simulink model "mchp_acim_dsPIC33A"  (R2025b)
settings: Solver=FixedStepDiscrete  StartTime=0.0  StopTime=25  FixedStep=Ts  RelTol=1e-3  EnableMultiTasking=on
values from neighbouring files (symbols this model uses):
  dataType = 'single'    [mchp_acim_foc_dsPIC33A_data.m]
  PWM_frequency = 20e3    (= 20000)    [mchp_acim_foc_dsPIC33A_data.m]
  PWM_frequency_mc = PWM_frequency    (= 20000)    [mchp_acim_foc_dsPIC33A_data.m]
  SpeedFilterCutoff = 40    [mchp_acim_foc_dsPIC33A_data.m]
  Ts = T_pwm    (= 5e-05)    [mchp_acim_foc_dsPIC33A_data.m]
  Ts_mc = T_pwm_mc    (= 5e-05)    [mchp_acim_foc_dsPIC33A_data.m]
  Ts_motor = T_pwm_mc    (= 5e-05)    [mchp_acim_foc_dsPIC33A_data.m]
  Ts_serialIn = 100e-3    (= 0.1)    [mchp_acim_foc_dsPIC33A_data.m]
undefined symbols (not defined in the file or in its folder): A0, A4, acim, ADC, appState, B0, C10, C11, C6, C7, C8, CS_param, D11, D12, DiscIntNeverNeededParam, estim_pll, estim_qei, inverter, Max, MaxPer, ms, NumBits1, NumBits2, P1, P17, P20, P39, P40, P41, P43, P44, P60, P61, PI_params_SI, Pin, PWM4_Trg1, Resol, s, target, us, VmaxPhase
libraries: simulink x47, MCHP_Blockset x24, mcbcontrolslib x5, mcbeeMathTransformLib x4, slpidlib x4, svdutilitieslib x1, autolibim x1, mcbplantlib x1
(part 6 of 6)

== system mchp_acim_dsPIC33A/Control algorithm/Motor Control Application/FOC/PI_Controller_Speed ==
  N_ref : Inport
  N_fb : Inport  Port=2
  Reset : Inport  Port=3
  Discrete PI Controller with anti-windup & reset : slpidlib/PID Controller  Controller=PI  Form=Parallel  TimeDomain=Discrete-time  UseExternalTs=off  SampleTime=Ts_mc  IntegratorMethod=Forward Euler  FilterMethod=Forward Euler  ControllerParametersSource=external  P=1  I=1  UseKiTs=on  D=0  UseExternalDerivativeSource=off  N=100  UseFilter=on  TunerSelectOption=Transfer Function Based (PID Tuner App)  InitialConditionSource=external  InitialConditionForIntegrator=0  InitialConditionForFilter=0  DifferentiatorICPrevScaledInput=0  ExternalReset=rising  TrackingMode=off  Kt=1  LimitOutput=on  SatLimitsSource=internal  UpperSaturationLimit=acim.Iq0  LowerSaturationLimit=-acim.Iq0  LinearizeAsGain=on  AntiWindupMode=clamping  Kb=1  LimitIntegrator=on  UpperIntegratorSaturationLimit=acim.Iq0  LowerIntegratorSaturationLimit=-acim.Iq0  RndMeth=Simplest  POutMin=[]  POutMax=[]  IOutMin=[]  IOutMax=[]  DOutMin=[]  DOutMax=[]  NOutMin=[]  NOutMax=[]  SumOutMin=[]  SumOutMax=[]  SaturationOutDataTypeStr=Inherit: Inherit via back propagation  SaturationOutMin=[]  SaturationOutMax=[]  PParamMin=[]  PParamMax=[]  IParamMin=[]  IParamMax=[]  DParamMin=[]  DParamMax=[]  NParamMin=[]  NParamMax=[]  KbParamMin=[]  KbParamMax=[]  KtParamMin=[]  KtParamMax=[]  KbOutMin=[]  KbOutMax=[]  KtOutMin=[]  KtOutMax=[]  IntegratorOutMin=[]  IntegratorOutMax=[]  FilterOutMin=[]  FilterOutMax=[]  SumI1OutMin=[]  SumI1OutMax=[]  SumI2OutMin=[]  SumI2OutMax=[]  SumI3OutMin=[]  SumI3OutMax=[]  SumI4OutMin=[]  SumI4OutMax=[]  SumDOutMin=[]  SumDOutMax=[]  DifferentiatorOutMin=[]  DifferentiatorOutMax=[]  FilterDiffOutCoefMin=[]  FilterDiffOutCoefMax=[]  ReciprocalOutMin=[]  ReciprocalOutMax=[]  SumDenOutMin=[]  SumDenOutMax=[]  SumNumOutMin=[]  SumNumOutMax=[]  DivideOutMin=[]  DivideOutMax=[]  UdiffTsProdOutMin=[]  UdiffTsProdOutMax=[]  NTsProdOutMin=[]  NTsProdOutMax=[]  UintegralTsProdOutMin=[]  UintegralTsProdOutMax=[]  UngainTsProdOutMin=[]  UngainTsProdOutMax=[]  ClampingZeroOutDataTypeStr=Inherit: Inherit via back propagation  ClampingZeroOutMin=[]  ClampingZeroOutMax=[]  FilterDenConstantOutDataTypeStr=Inherit: Inherit via back propagation  FilterDenConstantOutMin=[]  FilterDenConstantOutMax=[]  PCopyOutDataTypeStr=Inherit: Inherit via back propagation  PCopyOutMin=[]  PCopyOutMax=[]  NCopyOutDataTypeStr=Inherit: Inherit via back propagation  NCopyOutMin=[]  NCopyOutMax=[]  IntegratorContinuousStateAttributes=''  IntegratorStateMustResolveToSignalObject=off  IntegratorRTWStateStorageClass=Auto  FilterContinuousStateAttributes=''  FilterStateMustResolveToSignalObject=off  FilterRTWStateStorageClass=Auto  ParallelPVariant=ExternalParameters  IdealPVariant=Disabled  IVariant=ExternalParameters  DVariant=Disabled  IntegratorVariant=Discrete  SatVariant=Enabled  AWVariant=DiscClampingParallel  PCopyVariant=Disabled  TRVariant=Disabled  FdbkBlocksVariant=Forward  IdealPFdbkVariant=Disabled  SatFdbkVariant=Disabled  DerivativeFilterVariant=Disabled  NVariant=Disabled  NCopyVariant=Disabled_SignalSpec  FilterICVariant=Disabled  IntegratorICVariant=ExternalICs  ExternalResetVariant=ExternalReset  TRSumVariant=Passthrough  SumFdbkVariant=Disabled  SumVariant=Sum_PI  TsampFilterVariant=InternalTs  TsampNgainVariant=Passthrough  TsampIntegralVariant=Disabled_SignalSpec  ExternalSaturationOutDataTypeStr=Inherit: Same as second input  DerivativeSourceVariant=Disabled  PreIntVariant=InternalPreInt
  Ki1 : Constant  Value=PI_params_SI.Ki_speed*Ts_mc  OutDataTypeStr=single  SampleTime=Ts_mc
  Kp1 : Constant  Value=PI_params_SI.Kp_speed  OutDataTypeStr=single  SampleTime=Ts_mc
  Sum : Sum  Inputs=|+-  OutDataTypeStr=Inherit: Same as first input
  Iq_ref : Outport  VectorParamsAs1DForOutWhenUnconnected=off
  wires:
  N_ref/1 -> Sum/1
  [Integrator_PI_Speed] -> Discrete PI Controller with anti-windup & reset/5
  Reset/1 -> Discrete PI Controller with anti-windup & reset/4
  Sum/1 -> Discrete PI Controller with anti-windup & reset/1
  N_fb/1 -> Sum/2
  Kp1/1 -> Discrete PI Controller with anti-windup & reset/2
  Ki1/1 -> Discrete PI Controller with anti-windup & reset/3
  Discrete PI Controller with anti-windup & reset/1 -> Iq_ref/1

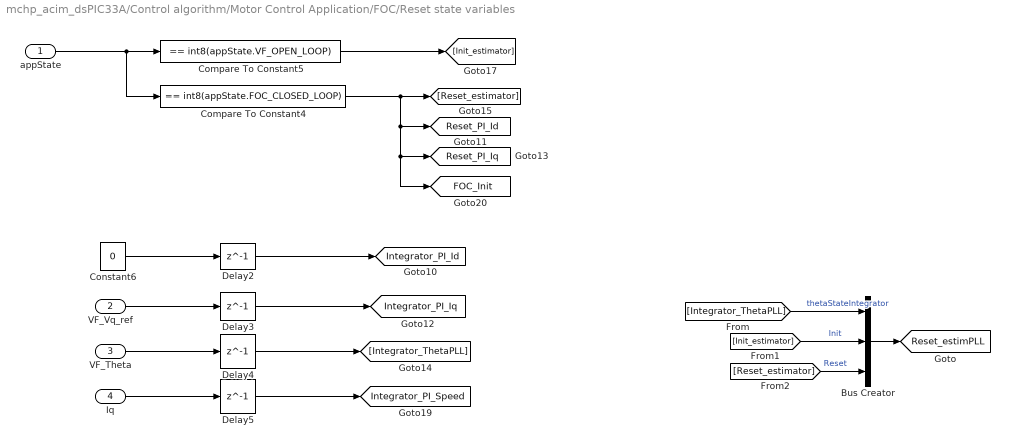
== system mchp_acim_dsPIC33A/Control algorithm/Motor Control Application/FOC/Reset state variables ==
  appState : Inport
  VF_Vq_ref : Inport  Port=2
  VF_Theta : Inport  Port=3
  Iq : Inport  Port=4
  Bus Creator : BusCreator  Inputs=3
  Compare To Constant4 : simulink/Logic and Bit Operations/Compare To Constant  relop===  const=int8(appState.FOC_CLOSED_LOOP)  OutDataTypeStr=boolean
  Compare To Constant5 : simulink/Logic and Bit Operations/Compare To Constant  relop===  const=int8(appState.VF_OPEN_LOOP)  OutDataTypeStr=boolean
  Constant6 : Constant  Value=0  OutDataTypeStr=single  SampleTime=-1
  Delay{2..5} (4 alike) : Delay  DelayLength=1
  tag scope: FOC_Init=global, Integrator_PI_Id=global, Integrator_PI_Iq=global, Integrator_PI_Speed=global, Reset_PI_Id=global, Reset_PI_Iq=global, Reset_estimPLL=global
  wires:
  Constant6/1 -> Delay2/1
  Compare To Constant4/1 -> [FOC_Init], [Reset_PI_Iq], [Reset_PI_Id], [Reset_estimator]
  Delay5/1 -> [Integrator_PI_Speed]
  Delay3/1 -> [Integrator_PI_Iq]
  Iq/1 -> Delay5/1
  appState/1 -> Compare To Constant4/1, Compare To Constant5/1
  VF_Theta/1 -> Delay4/1
  VF_Vq_ref/1 -> Delay3/1
  Delay2/1 -> [Integrator_PI_Id]
  Delay4/1 -> [Integrator_ThetaPLL]
  Compare To Constant5/1 -> [Init_estimator]
  [Integrator_ThetaPLL] -> Bus Creator/1  "thetaStateIntegrator"
  [Init_estimator] -> Bus Creator/2  "Init"
  [Reset_estimator] -> Bus Creator/3  "Reset"
  Bus Creator/1 -> [Reset_estimPLL]

== system mchp_acim_dsPIC33A/Control algorithm/Motor Control Application/FOC/VbyF ControlReference ==
  Reset : Inport
  speedRef : Inport  Port=2
  Enable : EnablePort
  Gain : Gain  Gain=(2*pi*acim.p/60)*Ts_mc  OutDataTypeStr=single
  Position Generator : mcbcontrolslib/Position Generator  AngleOutput=Radians  InitialThetaSource=Specify via dialog  ExternalReset=active high resets to initial condition  Offset=0
  Saturation : Saturate  UpperLimit=acim.V_rated*sqrt(2/3)*0.9  LowerLimit=10
  VbyF_constant : Gain  Gain=CS_param.VbyF_constant
  Wrap_to_pi1 : Subsystem  VariantControl=VSS_STD
  OL_Theta : Outport
  V_ref : Outport  Port=2
  wires:
  Gain/1 -> Position Generator/1
  Position Generator/1 -> Wrap_to_pi1/1(θ)  "Theta_in"
  Reset/1 -> Position Generator/2
  Wrap_to_pi1/1(θ (-π,π)) -> OL_Theta/1
  speedRef/1 -> VbyF_constant/1, Gain/1
  VbyF_constant/1 -> Saturation/1
  Saturation/1 -> V_ref/1

== system mchp_acim_dsPIC33A/Control algorithm/Motor Control Application/appState State Machine/Speed Ramp_limiter ==
  Reset_trigger : Inport
  Initial_value : Inport  Port=2
  Target_speed : Inport  Port=3
  stop : Inport  Port=4
  Compare To Constant2 : simulink/Logic and Bit Operations/Compare To Constant  relop=>=  const=CS_param.SpeedRampRate  OutDataTypeStr=boolean
  Compare To Constant7 : simulink/Logic and Bit Operations/Compare To Constant  relop=<=  const=-CS_param.SpeedRampRate  OutDataTypeStr=boolean
  Constant1 : Constant  Value=acim.N_min/2  OutDataTypeStr=single  SampleTime=-1
  Constant10 : Constant  Value=-CS_param.SpeedRampRate  OutDataTypeStr=single  SampleTime=-1
  Constant9 : Constant  Value=CS_param.SpeedRampRate  OutDataTypeStr=single  SampleTime=-1
  Delay1 : Delay  DelayLength=1  InitialConditionSource=Input port  InitialCondition=-1  ExternalReset=Level
      settings: InputPortMap=u0,r5,p4
  Product1 : Product
  Product3 : Product
  Subtract2 : Sum  Inputs=+-
  Subtract4 : Sum  Inputs=+++
  Switch : Switch  Criteria=u2 > Threshold  SaturateOnIntegerOverflow=off  InputSameDT=off
  Reference_Speed : Outport
  wires:
  Constant9/1 -> Product1/1
  Compare To Constant7/1 -> Product3/2
  Subtract2/1 -> Compare To Constant7/1, Compare To Constant2/1
  Delay1/1 -> Subtract2/2, Reference_Speed/1, Subtract4/1
  Constant10/1 -> Product3/1
  Compare To Constant2/1 -> Product1/2
  Subtract4/1 -> Delay1/1
  Product3/1 -> Subtract4/3
  Product1/1 -> Subtract4/2
  Reset_trigger/1 -> Delay1/2
  Switch/1 -> Subtract2/1
  Initial_value/1 -> Delay1/3
  stop/1 -> Switch/2
  Target_speed/1 -> Switch/3
  Constant1/1 -> Switch/1

== system mchp_acim_dsPIC33A/Inverter and Motor model/Simulation/Motor and Inverter/Inverter ==
  Duty_abc : Inport
  Average-Value Inverter : mcbplantlib/Average-Value Inverter
  Constant2 : Constant  Value=inverter.V_dc  OutDataTypeStr=single  SampleTime=-1
  Data Type Conversion1 : DataTypeConversion  OutDataTypeStr=single  RndMeth=Simplest  SaturateOnIntegerOverflow=off
  Vabc : Outport  VectorParamsAs1DForOutWhenUnconnected=off
  wires:
  Constant2/1 -> Average-Value Inverter/2
  Data Type Conversion1/1 -> Average-Value Inverter/1
  Duty_abc/1 -> Data Type Conversion1/1
  Average-Value Inverter/1 -> Vabc/1  "Vabc"

== system mchp_acim_dsPIC33A/MCHV-230VAC-1.5kW Development Board dsPIC33AK128MC106 MC DIM/Center & sign reversal1/Moving Average/Enabled Subsystem1 ==
  In1 : Inport
  Enable : EnablePort  ZeroCross=off
  Out1 : Outport
  wires:
  In1/1 -> Out1/1

== system mchp_acim_dsPIC33A/Control algorithm/Data Monitoring/SerialOutDrivers/codegen/SCI_Tx ==
  note: Fast Serial Data Monitoring (32-bit)
  Data_Log : Inport
  Constant : Constant  Value=target.frameSize -1  OutDataTypeStr=uint16
  Counter Limited : simulink/Sources/Counter Limited  uplimit=target.frameSize-1  tsamp=-1
  Data : Subsystem  TreatAsAtomicUnit=on
  Data Type Conversion : DataTypeConversion  OutDataTypeStr=uint16  RndMeth=Simplest  SaturateOnIntegerOverflow=off
  End : Subsystem  TreatAsAtomicUnit=on
  If : If  NumInputs=2  IfExpression=u1 == 0  ElseIfExpressions=u1 == u2
  Start : Subsystem  TreatAsAtomicUnit=on
  wires:
  If/3 -> Data/Action
  Counter Limited/1 -> Data Type Conversion/1
  If/2 -> End/Action
  If/1 -> Start/Action
  Data_Log/1 -> End/1(Data), Start/1(Data), Data/1(Data)
  Constant/1 -> If/2
  Data Type Conversion/1 -> If/1

== system mchp_acim_dsPIC33A/Control algorithm/Data Monitoring/Subsystem/Data_Conditioning_Tx/Data_Type_Fixed_Point ==
  In1 : Inport
  Data Type Conversion : DataTypeConversion  OutDataTypeStr=fixdt(1,32,28)  RndMeth=Simplest  SaturateOnIntegerOverflow=off
  Data Type Conversion3 : DataTypeConversion  OutDataTypeStr=uint32  ConvertRealWorld=Stored Integer (SI)  RndMeth=Simplest  SaturateOnIntegerOverflow=off
  Data_Log : Outport
  wires:
  In1/1 -> Data Type Conversion/1
  Data Type Conversion3/1 -> Data_Log/1
  Data Type Conversion/1 -> Data Type Conversion3/1

== system mchp_acim_dsPIC33A/Control algorithm/Data Monitoring/Subsystem/Data_Conditioning_Tx/Data_Type_Float ==
  In1 : Inport
  Byte Pack : svdutilitieslib/Byte Pack  maskPackedDataType=uint8  datatypes={'single'}  byteAlign=4  blockPlatform=tic2000
  Data_Log : Outport
  wires:
  Byte Pack/1 -> Data_Log/1
  In1/1 -> Byte Pack/1

== system mchp_acim_dsPIC33A/Control algorithm/Data Monitoring/Variant Subsystem/Codegen/Extract User inputs ==
  SCi_Data : Inport
  Bitwise OR : simulink/Logic and Bit Operations/Bitwise Operator  logicop=OR  UseBitMask=off  NumInputPorts=2  BitMask=bin2dec('11011001')  BitMaskRealWorld=Stored Integer
  Data Type Conversion1 : DataTypeConversion  OutDataTypeStr=uint16  RndMeth=Simplest  SaturateOnIntegerOverflow=off
  Data Type Conversion2 : DataTypeConversion  OutDataTypeStr=int16  ConvertRealWorld=Stored Integer (SI)  RndMeth=Simplest  SaturateOnIntegerOverflow=off
  Data Type Conversion3 : DataTypeConversion  OutDataTypeStr=uint16  RndMeth=Simplest  SaturateOnIntegerOverflow=off
  Data Type Conversion4 : DataTypeConversion  OutDataTypeStr=dataType  RndMeth=Simplest  SaturateOnIntegerOverflow=off
  Demux : Demux  Outputs=8
  RPM to rad/s : Gain  Gain=pi/30  RndMeth=Simplest  OutDataTypeStr=Inherit: Same as input
  Shift Arithmetic : ArithShift  BitShiftNumber=-8
  Terminator{,1..3} (4 alike) : Terminator
  Enable : Outport
  SpeedRef : Outport  Port=2
  DebugSel : Outport  Port=3
  wires:
  Demux/3 -> Enable/1
  Data Type Conversion2/1 -> Data Type Conversion4/1  "SpeedRef"
  Demux/4 -> DebugSel/1
  Bitwise OR/1 -> Data Type Conversion2/1
  Demux/1 -> Data Type Conversion1/1
  SCi_Data/1 -> Demux/1
  Shift Arithmetic/1 -> Bitwise OR/2
  Data Type Conversion3/1 -> Shift Arithmetic/1
  Data Type Conversion1/1 -> Bitwise OR/1
  Demux/7 -> Terminator2/1
  Demux/2 -> Data Type Conversion3/1
  Demux/5 -> Terminator/1
  Demux/6 -> Terminator1/1
  Demux/8 -> Terminator3/1
  RPM to rad/s/1 -> SpeedRef/1  "SpeedRef"
  Data Type Conversion4/1 -> RPM to rad/s/1

== system mchp_acim_dsPIC33A/Control algorithm/Motor Control Application/FOC/Current_Controllers/Dynamic Limit ==
  Vd : Inport
  Constant : Constant  Value=CS_param.VmaxPhase  OutDataTypeStr=single  SampleTime=-1
  Product : Product  RndMeth=Simplest  OutDataTypeStr=Inherit: Same as first input
  Product1 : Product  RndMeth=Simplest  OutDataTypeStr=Inherit: Same as first input
  Saturation : Saturate  UpperLimit=CS_param.VmaxPhase^2  LowerLimit=0
  Sqrt : Sqrt  RndMeth=Simplest
  Sum1 : Sum  Inputs=+-|  RndMeth=Simplest  OutDataTypeStr=Inherit: Same as first input
  Vq_max : Outport
  wires:
  Vd/1 -> Product/1, Product/2
  Product/1 -> Saturation/1
  Constant/1 -> Product1/2, Product1/1
  Saturation/1 -> Sum1/2
  Sum1/1 -> Sqrt/1
  Product1/1 -> Sum1/1
  Sqrt/1 -> Vq_max/1

== system mchp_acim_dsPIC33A/Control algorithm/Motor Control Application/FOC/Current_Controllers/PI_Controller_Id ==
  I_ref : Inport
  I_fb : Inport  Port=2
  Discrete PI Controller with anti-windup & reset : slpidlib/PID Controller  Controller=PI  Form=Parallel  TimeDomain=Discrete-time  UseExternalTs=off  SampleTime=Ts_mc  IntegratorMethod=Forward Euler  FilterMethod=Forward Euler  ControllerParametersSource=external  P=1  I=1  UseKiTs=on  D=0  UseExternalDerivativeSource=off  N=100  UseFilter=on  TunerSelectOption=Transfer Function Based (PID Tuner App)  InitialConditionSource=external  InitialConditionForIntegrator=0  InitialConditionForFilter=0  DifferentiatorICPrevScaledInput=0  ExternalReset=rising  TrackingMode=off  Kt=1  LimitOutput=on  SatLimitsSource=internal  UpperSaturationLimit=CS_param.VmaxPhase  LowerSaturationLimit=-CS_param.VmaxPhase  LinearizeAsGain=on  AntiWindupMode=clamping  Kb=1  LimitIntegrator=on  UpperIntegratorSaturationLimit=CS_param.VmaxPhase  LowerIntegratorSaturationLimit=-CS_param.VmaxPhase  RndMeth=Simplest  POutMin=[]  POutMax=[]  IOutMin=[]  IOutMax=[]  DOutMin=[]  DOutMax=[]  NOutMin=[]  NOutMax=[]  SumOutMin=[]  SumOutMax=[]  SaturationOutDataTypeStr=Inherit: Inherit via back propagation  SaturationOutMin=[]  SaturationOutMax=[]  PParamMin=[]  PParamMax=[]  IParamMin=[]  IParamMax=[]  DParamMin=[]  DParamMax=[]  NParamMin=[]  NParamMax=[]  KbParamMin=[]  KbParamMax=[]  KtParamMin=[]  KtParamMax=[]  KbOutMin=[]  KbOutMax=[]  KtOutMin=[]  KtOutMax=[]  IntegratorOutMin=[]  IntegratorOutMax=[]  FilterOutMin=[]  FilterOutMax=[]  SumI1OutMin=[]  SumI1OutMax=[]  SumI2OutMin=[]  SumI2OutMax=[]  SumI3OutMin=[]  SumI3OutMax=[]  SumI4OutMin=[]  SumI4OutMax=[]  SumDOutMin=[]  SumDOutMax=[]  DifferentiatorOutMin=[]  DifferentiatorOutMax=[]  FilterDiffOutCoefMin=[]  FilterDiffOutCoefMax=[]  ReciprocalOutMin=[]  ReciprocalOutMax=[]  SumDenOutMin=[]  SumDenOutMax=[]  SumNumOutMin=[]  SumNumOutMax=[]  DivideOutMin=[]  DivideOutMax=[]  UdiffTsProdOutMin=[]  UdiffTsProdOutMax=[]  NTsProdOutMin=[]  NTsProdOutMax=[]  UintegralTsProdOutMin=[]  UintegralTsProdOutMax=[]  UngainTsProdOutMin=[]  UngainTsProdOutMax=[]  ClampingZeroOutDataTypeStr=Inherit: Inherit via back propagation  ClampingZeroOutMin=[]  ClampingZeroOutMax=[]  FilterDenConstantOutDataTypeStr=Inherit: Inherit via back propagation  FilterDenConstantOutMin=[]  FilterDenConstantOutMax=[]  PCopyOutDataTypeStr=Inherit: Inherit via back propagation  PCopyOutMin=[]  PCopyOutMax=[]  NCopyOutDataTypeStr=Inherit: Inherit via back propagation  NCopyOutMin=[]  NCopyOutMax=[]  IntegratorContinuousStateAttributes=''  IntegratorStateMustResolveToSignalObject=off  IntegratorRTWStateStorageClass=Auto  FilterContinuousStateAttributes=''  FilterStateMustResolveToSignalObject=off  FilterRTWStateStorageClass=Auto  ParallelPVariant=ExternalParameters  IdealPVariant=Disabled  IVariant=ExternalParameters  DVariant=Disabled  IntegratorVariant=Discrete  SatVariant=Enabled  AWVariant=DiscClampingParallel  PCopyVariant=Disabled  TRVariant=Disabled  FdbkBlocksVariant=Forward  IdealPFdbkVariant=Disabled  SatFdbkVariant=Disabled  DerivativeFilterVariant=Disabled  NVariant=Disabled  NCopyVariant=Disabled_SignalSpec  FilterICVariant=Disabled  IntegratorICVariant=ExternalICs  ExternalResetVariant=ExternalReset  TRSumVariant=Passthrough  SumFdbkVariant=Disabled  SumVariant=Sum_PI  TsampFilterVariant=InternalTs  TsampNgainVariant=Passthrough  TsampIntegralVariant=Disabled_SignalSpec  ExternalSaturationOutDataTypeStr=Inherit: Same as second input  DerivativeSourceVariant=Disabled  PreIntVariant=InternalPreInt
  Ki3 : Constant  Value=PI_params_SI.Ki_i*Ts_mc  OutDataTypeStr=single  SampleTime=Ts_mc
  Kp2 : Constant  Value=PI_params_SI.Kp_i  OutDataTypeStr=single  SampleTime=Ts_mc
  Sum : Sum  Inputs=|+-  OutDataTypeStr=Inherit: Same as first input
  V_ref : Outport  VectorParamsAs1DForOutWhenUnconnected=off
  wires:
  [Integrator_PI_Id] -> Discrete PI Controller with anti-windup & reset/5
  Sum/1 -> Discrete PI Controller with anti-windup & reset/1
  Discrete PI Controller with anti-windup & reset/1 -> V_ref/1
  I_fb/1 -> Sum/2
  I_ref/1 -> Sum/1
  Ki3/1 -> Discrete PI Controller with anti-windup & reset/3
  Kp2/1 -> Discrete PI Controller with anti-windup & reset/2
  [Reset_PI_Id] -> Discrete PI Controller with anti-windup & reset/4

== system mchp_acim_dsPIC33A/Control algorithm/Motor Control Application/FOC/Current_Controllers/PI_Controller_Iq ==
  I_ref : Inport
  I_fb : Inport  Port=2
  Vq_max : Inport  Port=3
  Discrete PI Controller with anti-windup & reset : slpidlib/PID Controller  Controller=PI  Form=Parallel  TimeDomain=Discrete-time  UseExternalTs=off  SampleTime=Ts_mc  IntegratorMethod=Forward Euler  FilterMethod=Forward Euler  ControllerParametersSource=external  P=1  I=1  UseKiTs=on  D=0  UseExternalDerivativeSource=off  N=100  UseFilter=on  TunerSelectOption=Transfer Function Based (PID Tuner App)  InitialConditionSource=external  InitialConditionForIntegrator=0  InitialConditionForFilter=0  DifferentiatorICPrevScaledInput=0  ExternalReset=rising  TrackingMode=off  Kt=1  LimitOutput=on  SatLimitsSource=external  UpperSaturationLimit=VmaxPhase  LowerSaturationLimit=-VmaxPhase  LinearizeAsGain=on  AntiWindupMode=clamping  Kb=1  LimitIntegrator=on  UpperIntegratorSaturationLimit=CS_param.VmaxPhase  LowerIntegratorSaturationLimit=-CS_param.VmaxPhase  RndMeth=Simplest  POutMin=[]  POutMax=[]  IOutMin=[]  IOutMax=[]  DOutMin=[]  DOutMax=[]  NOutMin=[]  NOutMax=[]  SumOutMin=[]  SumOutMax=[]  SaturationOutDataTypeStr=Inherit: Inherit via back propagation  SaturationOutMin=[]  SaturationOutMax=[]  PParamMin=[]  PParamMax=[]  IParamMin=[]  IParamMax=[]  DParamMin=[]  DParamMax=[]  NParamMin=[]  NParamMax=[]  KbParamMin=[]  KbParamMax=[]  KtParamMin=[]  KtParamMax=[]  KbOutMin=[]  KbOutMax=[]  KtOutMin=[]  KtOutMax=[]  IntegratorOutMin=[]  IntegratorOutMax=[]  FilterOutMin=[]  FilterOutMax=[]  SumI1OutMin=[]  SumI1OutMax=[]  SumI2OutMin=[]  SumI2OutMax=[]  SumI3OutMin=[]  SumI3OutMax=[]  SumI4OutMin=[]  SumI4OutMax=[]  SumDOutMin=[]  SumDOutMax=[]  DifferentiatorOutMin=[]  DifferentiatorOutMax=[]  FilterDiffOutCoefMin=[]  FilterDiffOutCoefMax=[]  ReciprocalOutMin=[]  ReciprocalOutMax=[]  SumDenOutMin=[]  SumDenOutMax=[]  SumNumOutMin=[]  SumNumOutMax=[]  DivideOutMin=[]  DivideOutMax=[]  UdiffTsProdOutMin=[]  UdiffTsProdOutMax=[]  NTsProdOutMin=[]  NTsProdOutMax=[]  UintegralTsProdOutMin=[]  UintegralTsProdOutMax=[]  UngainTsProdOutMin=[]  UngainTsProdOutMax=[]  ClampingZeroOutDataTypeStr=Inherit: Inherit via back propagation  ClampingZeroOutMin=[]  ClampingZeroOutMax=[]  FilterDenConstantOutDataTypeStr=Inherit: Inherit via back propagation  FilterDenConstantOutMin=[]  FilterDenConstantOutMax=[]  PCopyOutDataTypeStr=Inherit: Inherit via back propagation  PCopyOutMin=[]  PCopyOutMax=[]  NCopyOutDataTypeStr=Inherit: Inherit via back propagation  NCopyOutMin=[]  NCopyOutMax=[]  IntegratorContinuousStateAttributes=''  IntegratorStateMustResolveToSignalObject=off  IntegratorRTWStateStorageClass=Auto  FilterContinuousStateAttributes=''  FilterStateMustResolveToSignalObject=off  FilterRTWStateStorageClass=Auto  ParallelPVariant=ExternalParameters  IdealPVariant=Disabled  IVariant=ExternalParameters  DVariant=Disabled  IntegratorVariant=Discrete  SatVariant=External  AWVariant=DiscClampingParallel  PCopyVariant=Disabled  TRVariant=Disabled  FdbkBlocksVariant=Forward  IdealPFdbkVariant=Disabled  SatFdbkVariant=Disabled  DerivativeFilterVariant=Disabled  NVariant=Disabled  NCopyVariant=Disabled_SignalSpec  FilterICVariant=Disabled  IntegratorICVariant=ExternalICs  ExternalResetVariant=ExternalReset  TRSumVariant=Passthrough  SumFdbkVariant=Disabled  SumVariant=Sum_PI  TsampFilterVariant=InternalTs  TsampNgainVariant=Passthrough  TsampIntegralVariant=Disabled_SignalSpec  ExternalSaturationOutDataTypeStr=Inherit: Same as second input  DerivativeSourceVariant=Disabled  PreIntVariant=InternalPreInt
  Gain : Gain  Gain=-1
  Ki3 : Constant  Value=PI_params_SI.Ki_i*Ts_mc  OutDataTypeStr=single  SampleTime=Ts_mc
  Kp2 : Constant  Value=PI_params_SI.Kp_i  OutDataTypeStr=single  SampleTime=Ts_mc
  Sum : Sum  Inputs=|+-  OutDataTypeStr=Inherit: Same as first input
  V_ref : Outport  VectorParamsAs1DForOutWhenUnconnected=off
  wires:
  [Integrator_PI_Iq] -> Discrete PI Controller with anti-windup & reset/5
  Sum/1 -> Discrete PI Controller with anti-windup & reset/1
  I_ref/1 -> Sum/1
  I_fb/1 -> Sum/2
  Discrete PI Controller with anti-windup & reset/1 -> V_ref/1
  [Reset_PI_Iq] -> Discrete PI Controller with anti-windup & reset/4
  Kp2/1 -> Discrete PI Controller with anti-windup & reset/2
  Ki3/1 -> Discrete PI Controller with anti-windup & reset/3
  Gain/1 -> Discrete PI Controller with anti-windup & reset/7
  Vq_max/1 -> Discrete PI Controller with anti-windup & reset/6, Gain/1

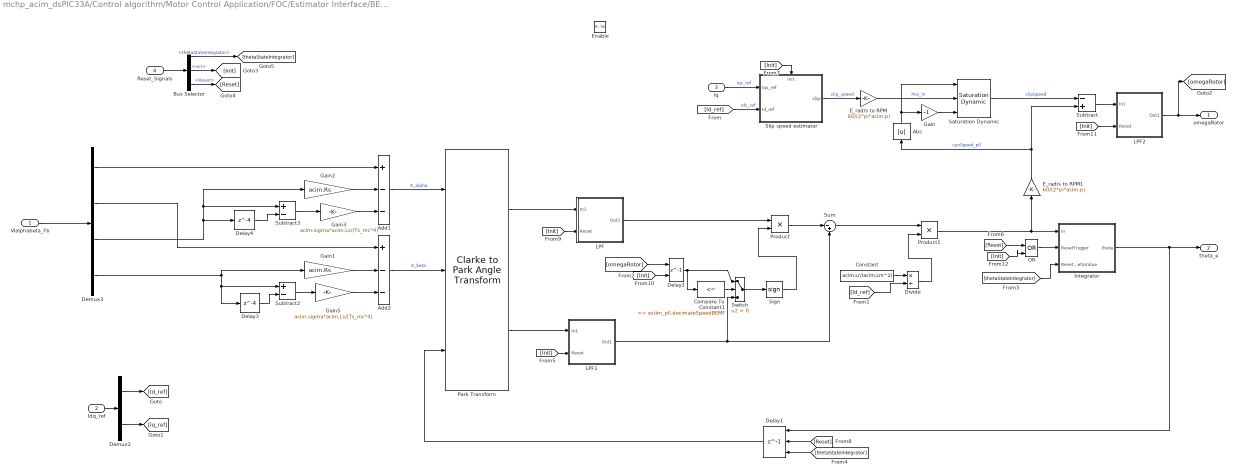
== system mchp_acim_dsPIC33A/Control algorithm/Motor Control Application/FOC/Estimator Interface/BEMF-PLL Sensorless estimator1 ==
  VIalphabeta_Fb : Inport
  Idq_ref : Inport  Port=2
  Iq : Inport  Port=3
  Reset_Signals : Inport  Port=4
  Enable : EnablePort
  Abs : Abs  SaturateOnIntegerOverflow=off
  Add1 : Sum  Inputs=+--
  Add2 : Sum  Inputs=+--
  Bus Selector : BusSelector  OutputSignals=thetaStateIntegrator,Init,Reset
  Compare To Constant1 : simulink/Logic and Bit Operations/Compare To Constant  relop=<=  const=estim_pll.decimateSpeedBEMF  OutDataTypeStr=boolean
  Constant : Constant  Value=acim.Lr/(acim.Lm^2)  OutDataTypeStr=single  SampleTime=-1
  Delay1 : Delay  DelayLength=1  InitialConditionSource=Input port  ExternalReset=Rising
      settings: InputPortMap=u0,r5,p4
  Delay2 : Delay  DelayLength=1  ExternalReset=Rising
      settings: InputPortMap=u0,r5
  Delay3 : Delay  DelayLength=4
  Delay4 : Delay  DelayLength=4
  Demux2 : Demux  Outputs=2
  Demux3 : Demux
  Divide : Product  Inputs=*/
  E_rad/s to RPM : Gain  Gain=60/(2*pi*acim.p)  RndMeth=Simplest  OutDataTypeStr=Inherit: Same as input
  E_rad/s to RPM1 : Gain  Gain=60/(2*pi*acim.p)  RndMeth=Simplest  OutDataTypeStr=Inherit: Same as input
  Gain : Gain  Gain=-1
  Gain1 : Gain  Gain=acim.Rs  OutDataTypeStr=Inherit: Same as input
  Gain2 : Gain  Gain=acim.Rs  OutDataTypeStr=Inherit: Same as input
  Gain3 : Gain  Gain=acim.sigma*acim.Ls/(Ts_mc*4)  OutDataTypeStr=single
  Gain5 : Gain  Gain=acim.sigma*acim.Ls/(Ts_mc*4)  OutDataTypeStr=single
  Integrator : Subsystem
  LPF : Subsystem
  LPF1 : Subsystem
  LPF2 : Subsystem
  OR : Logic  Operator=OR  IconShape=distinctive  AllPortsSameDT=off  OutDataTypeStr=boolean
  Park Transform : mcbeeMathTransformLib/Clarke to Park Angle Transform  AxisAlignment=D-axis  UseWithEmbedded=on  PhaseInput=Two inputs  ThetaInput=Electrical position  AngleInput=Radians  N_points=1024
      settings: LibrarySourceBlock=mcbcontrolslib/Park Transform
  Product : Product
  Product1 : Product
  Saturation Dynamic : simulink/Discontinuities/Saturation Dynamic  OutMin=[]  OutMax=[]  OutDataTypeStr=Inherit: Same as second input  OutDataType=fixdt(1, 16)  OutScaling=2^-10  DoSatur=off
  Sign : Signum
  Slip speed estimator : Subsystem
      settings: PortSchema="{\"entries\":[{\"content\":{\"sides\":[{\"content\":{\"connectorIds\":[\"In1\",\"In2\"]},\"type\":\"ConnectorPlacement.EquallySpacedRectSide\",\"uuid\":\"981370cc-fd81-43b0-8526-c66c0de54492\"},{\"content\":{\"connectorIds\":[\"Out1\"],\"side\":\"RIGHT\"},\"type\":\"ConnectorPlacement.EquallySpacedRectSide\",\"uuid\":\"4a494ed1-db1f-498e-bde6-92ddc00b959f\"},{\"content\":{\"connectorIds\":[\"In3\"],\"side\":\"TOP\"},\"type\":\"ConnectorPlacement.EquallySpacedRectSide\",\"uuid\":\"ae0cfd30-3876-4cea-9557-00c7dbe354cc\"}]},\"type\":\"ConnectorPlacement.EquallySpacedConnector\",\"uuid\":\"0c170fee-798a-45d3-abb0-c7a31b583370\"}],\"packageUris\":[\"http://schema.mathworks.com/mf0/Connector/R2020b\"],\"version\":\"1.0\"}"
  Subtract : Sum  Inputs=-+
  Subtract2 : Sum  Inputs=+-
  Subtract3 : Sum  Inputs=+-
  Sum : Sum  Inputs=|-+
  Switch : Switch  Criteria=u2 > Threshold  SaturateOnIntegerOverflow=off  InputSameDT=off
  omegaRotor : Outport
  theta_e : Outport  Port=2
  wires:
  Sign/1 -> Product/2
  Sum/1 -> Product1/1
  Delay1/1 -> Park Transform/3
  Add2/1 -> Park Transform/2  "E_beta"
  Product/1 -> Sum/1
  VIalphabeta_Fb/1 -> Demux3/1
  Add1/1 -> Park Transform/1  "E_alpha"
  Park Transform/1 -> LPF/1(In1)
  LPF/1(Out1) -> Product/1
  Park Transform/2 -> LPF1/1(In1)
  Integrator/1(theta) -> Delay1/1, theta_e/1
  Idq_ref/1 -> Demux2/1
  Demux2/1 -> [Id_ref]
  Demux2/2 -> [Iq_ref]
  Constant/1 -> Divide/1
  [Id_ref] -> Divide/2
  Divide/1 -> Product1/2
  Iq/1 -> Slip speed estimator/1(Iqs_ref)  "Iqs_ref"
  Slip speed estimator/1(slip) -> E_rad/s to RPM/1  "slip_speed"
  E_rad/s to RPM/1 -> Saturation Dynamic/2  "Pos_In"
  Product1/1 -> Integrator/1(In), E_rad/s to RPM1/1
  LPF2/1(Out1) -> [omegaRotor], omegaRotor/1
  E_rad/s to RPM1/1 -> Abs/1, Subtract/2  "synSpeed_pll"
  Gain/1 -> Saturation Dynamic/3
  Saturation Dynamic/1 -> Subtract/1  "slipSpeed"
  Compare To Constant1/1 -> Switch/2
  Delay2/1 -> Compare To Constant1/1, Switch/1
  LPF1/1(Out1) -> Switch/3, Sum/2
  Switch/1 -> Sign/1
  OR/1 -> Integrator/2(ResetTrigger)
  [Id_ref] -> Slip speed estimator/2(Id_ref)  "Ids_ref"
  Abs/1 -> Saturation Dynamic/1, Gain/1
  Subtract/1 -> LPF2/1(In1)
  Demux3/1 -> Add1/1
  Demux3/3 -> Delay4/1, Gain2/1, Subtract3/1
  Subtract3/1 -> Gain3/1
  Delay4/1 -> Subtract3/2
  Gain2/1 -> Add1/2
  Gain3/1 -> Add1/3
  Gain5/1 -> Add2/3
  Delay3/1 -> Subtract2/2
  Subtract2/1 -> Gain5/1
  Demux3/2 -> Add2/1
  Demux3/4 -> Gain1/1, Subtract2/1, Delay3/1
  Gain1/1 -> Add2/2
  [omegaRotor] -> Delay2/1
  [Reset] -> OR/1
  [Init] -> OR/2
  Reset_Signals/1 -> Bus Selector/1
  Bus Selector/2 -> [Init]  "<Init>"
  Bus Selector/3 -> [Reset]  "<Reset>"
  Bus Selector/1 -> [thetaStateIntegrator]  "<thetaStateIntegrator>"
  [thetaStateIntegrator] -> Integrator/3(ResetThetaValue)
  [thetaStateIntegrator] -> Delay1/3
  [Reset] -> Delay1/2
  [Init] -> LPF1/2(Reset)
  [Init] -> LPF/2(Reset)
  [Init] -> Delay2/2
  [Init] -> LPF2/2(Reset)
  [Init] -> Slip speed estimator/3(Init)

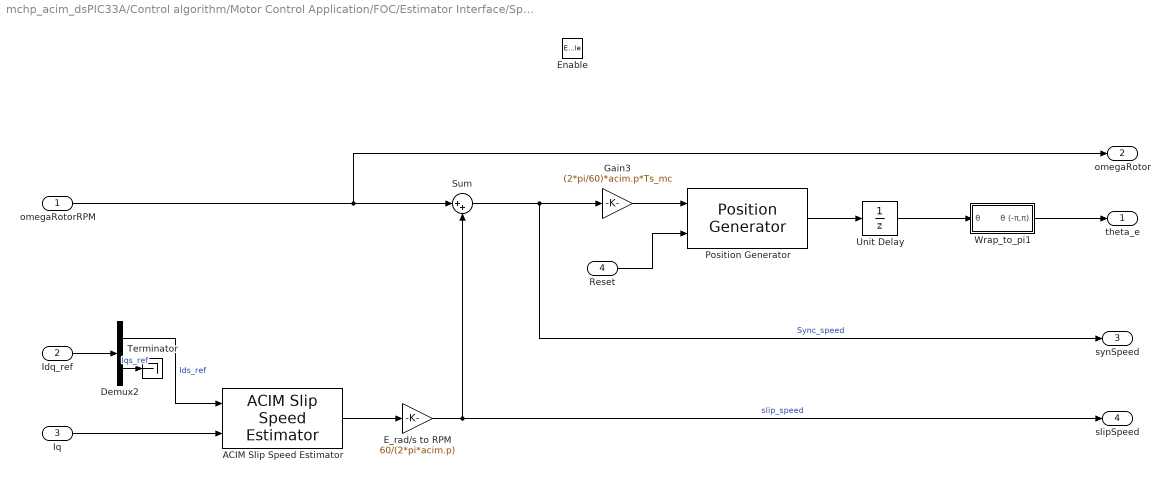
== system mchp_acim_dsPIC33A/Control algorithm/Motor Control Application/FOC/Estimator Interface/Speed & postion interface (sensored) ==
  omegaRotorRPM : Inport
  Idq_ref : Inport  Port=2
  Iq : Inport  Port=3
  Reset : Inport  Port=4
  Enable : EnablePort
  ACIM Slip Speed Estimator : mcbcontrolslib/ACIM Slip Speed Estimator  polePairs=acim.p  Rr=acim.Rr  Llr=acim.Llr  Lm=acim.Lm  N_sat=acim.N_rated/20  Units=SI Units  N_base=acim.N_base
  Demux2 : Demux  Outputs=2
  E_rad/s to RPM : Gain  Gain=60/(2*pi*acim.p)  RndMeth=Simplest  OutDataTypeStr=Inherit: Same as input
  Gain3 : Gain  Gain=(2*pi/60)*acim.p*Ts_mc  RndMeth=Simplest  OutDataTypeStr=Inherit: Same as input
  Position Generator : mcbcontrolslib/Position Generator  AngleOutput=Radians  InitialThetaSource=Specify via dialog  ExternalReset=active high resets to initial condition  Offset=0
  Sum : Sum  Inputs=|++
  Terminator : Terminator
  Unit Delay : UnitDelay  SampleTime=-1  HasFrameUpgradeWarning=on
  Wrap_to_pi1 : Subsystem  VariantControl=VSS_STD
  theta_e : Outport
  omegaRotor : Outport  Port=2
  synSpeed : Outport  Port=3
  slipSpeed : Outport  Port=4
  wires:
  Position Generator/1 -> Unit Delay/1
  Sum/1 -> synSpeed/1, Gain3/1  "Sync_speed"
  Demux2/1 -> ACIM Slip Speed Estimator/1  "Ids_ref"
  ACIM Slip Speed Estimator/1 -> E_rad/s to RPM/1
  Gain3/1 -> Position Generator/1
  Reset/1 -> Position Generator/2
  Idq_ref/1 -> Demux2/1
  Unit Delay/1 -> Wrap_to_pi1/1(θ)
  omegaRotorRPM/1 -> omegaRotor/1, Sum/1
  E_rad/s to RPM/1 -> Sum/2, slipSpeed/1  "slip_speed"
  Wrap_to_pi1/1(θ (-π,π)) -> theta_e/1
  Iq/1 -> ACIM Slip Speed Estimator/2
  Demux2/2 -> Terminator/1  "Iqs_ref"

== system mchp_acim_dsPIC33A/Control algorithm/Motor Control Application/FOC/Generate Id reference/Enabled Subsystem ==
  In1 : Inport
  Enable : EnablePort
  Out1 : Outport
  wires:
  In1/1 -> Out1/1

== system mchp_acim_dsPIC33A/Control algorithm/Motor Control Application/FOC/Generate Id reference/Inverse Speed based Flux Weakening ==
  SpeedRef : Inport
  Enable : EnablePort
  Compare To Constant : simulink/Logic and Bit Operations/Compare To Constant  relop=>=  const=acim.N_rated/2  OutDataTypeStr=uint8
  If : If  IfExpression=(u1 > 0)
  If Action Subsystem : Subsystem  TreatAsAtomicUnit=on
  If Action Subsystem1 : Subsystem  TreatAsAtomicUnit=on
  Merge : Merge
  Id_ref : Outport
  wires:
  SpeedRef/1 -> If Action Subsystem/1(speedRef), Compare To Constant/1
  Compare To Constant/1 -> If/1
  If Action Subsystem/1(id_ref) -> Merge/1
  If/1 -> If Action Subsystem/Action
  If/2 -> If Action Subsystem1/Action
  If Action Subsystem1/1(id_ref) -> Merge/2
  Merge/1 -> Id_ref/1

== system mchp_acim_dsPIC33A/Control algorithm/Motor Control Application/FOC/Generate Id reference/OffsetRamp ==
  In1 : Inport
  In2 : Inport  Port=2
  Abs2 : Abs  SaturateOnIntegerOverflow=off
  Compare To Constant6 : simulink/Logic and Bit Operations/Compare To Constant  relop=<=  const=CS_param.currentRampRate  OutDataTypeStr=boolean
  Constant14 : Constant  Value=CS_param.currentRampRate  OutDataTypeStr=single
  Constant6 : Constant  Value=0  OutDataTypeStr=single
  Delay : Delay  DelayLength=1  InitialConditionSource=Input port  InitialCondition=-1  ExternalReset=Rising
      settings: InputPortMap=u0,r5,p4
  Product2 : Product
  Sign2 : Signum
  Subtract3 : Sum  Inputs=+-  OutDataTypeStr=single  AccumDataTypeStr=single
  Switch1 : Switch  Criteria=u2 > Threshold  SaturateOnIntegerOverflow=off  InputSameDT=off
  Out1 : Outport
  wires:
  Subtract3/1 -> Delay/1, Switch1/3, Abs2/1
  Constant6/1 -> Switch1/1
  Sign2/1 -> Product2/1
  Delay/1 -> Sign2/1, Subtract3/1
  Abs2/1 -> Compare To Constant6/1
  Product2/1 -> Subtract3/2
  Constant14/1 -> Product2/2
  Compare To Constant6/1 -> Switch1/2
  Switch1/1 -> Out1/1
  In1/1 -> Delay/2
  In2/1 -> Delay/3

== system mchp_acim_dsPIC33A/Control algorithm/Motor Control Application/FOC/Generate Id reference/Voltage limit based Flux Weakening ==
  SpeedRef : Inport
  vdq : Inport  Port=2
  Enable : EnablePort
  Add1 : Sum
  Compare To Constant : simulink/Logic and Bit Operations/Compare To Constant  relop=<=  const=acim.N_rated/2  OutDataTypeStr=boolean
  Constant : Constant  Value=CS_param.VmaxPhase*0.9  OutDataTypeStr=single
  Delay One Step : Delay  DelayLength=1
  Demux : Demux  Outputs=2
  Discrete PID Controller : slpidlib/PID Controller  Controller=PI  Form=Parallel  TimeDomain=Discrete-time  UseExternalTs=off  SampleTime=-1  IntegratorMethod=Forward Euler  FilterMethod=Forward Euler  ControllerParametersSource=internal  P=PI_params_SI.Kp_FW  I=PI_params_SI.Ki_FW  UseKiTs=on  D=0  UseExternalDerivativeSource=off  N=100  UseFilter=on  TunerSelectOption=Transfer Function Based (PID Tuner App)  InitialConditionSource=internal  InitialConditionForIntegrator=acim.Id0  InitialConditionForFilter=0  DifferentiatorICPrevScaledInput=0  ExternalReset=level  TrackingMode=off  Kt=1  LimitOutput=on  SatLimitsSource=internal  UpperSaturationLimit=acim.Id0  LowerSaturationLimit=acim.Id0/2  LinearizeAsGain=off  AntiWindupMode=none  Kb=1  LimitIntegrator=on  UpperIntegratorSaturationLimit=acim.Id0  LowerIntegratorSaturationLimit=acim.Id0/2  POutMin=[]  POutMax=[]  IOutMin=[]  IOutMax=[]  DOutMin=[]  DOutMax=[]  NOutMin=[]  NOutMax=[]  SumOutMin=[]  SumOutMax=[]  SaturationOutMin=[]  SaturationOutMax=[]  PParamMin=[]  PParamMax=[]  IParamMin=[]  IParamMax=[]  DParamMin=[]  DParamMax=[]  NParamMin=[]  NParamMax=[]  KbParamMin=[]  KbParamMax=[]  KtParamMin=[]  KtParamMax=[]  KbOutMin=[]  KbOutMax=[]  KtOutMin=[]  KtOutMax=[]  IntegratorOutMin=[]  IntegratorOutMax=[]  FilterOutMin=[]  FilterOutMax=[]  SumI1OutMin=[]  SumI1OutMax=[]  SumI2OutMin=[]  SumI2OutMax=[]  SumI3OutMin=[]  SumI3OutMax=[]  SumI4OutMin=[]  SumI4OutMax=[]  SumDOutMin=[]  SumDOutMax=[]  DifferentiatorOutMin=[]  DifferentiatorOutMax=[]  FilterDiffOutCoefMin=[]  FilterDiffOutCoefMax=[]  ReciprocalOutMin=[]  ReciprocalOutMax=[]  SumDenOutMin=[]  SumDenOutMax=[]  SumNumOutMin=[]  SumNumOutMax=[]  DivideOutMin=[]  DivideOutMax=[]  UdiffTsProdOutMin=[]  UdiffTsProdOutMax=[]  NTsProdOutMin=[]  NTsProdOutMax=[]  UintegralTsProdOutMin=[]  UintegralTsProdOutMax=[]  UngainTsProdOutMin=[]  UngainTsProdOutMax=[]  ClampingZeroOutDataTypeStr=Inherit: Inherit via back propagation  ClampingZeroOutMin=[]  ClampingZeroOutMax=[]  FilterDenConstantOutDataTypeStr=Inherit: Inherit via back propagation  FilterDenConstantOutMin=[]  FilterDenConstantOutMax=[]  PCopyOutDataTypeStr=Inherit: Inherit via back propagation  PCopyOutMin=[]  PCopyOutMax=[]  NCopyOutDataTypeStr=Inherit: Inherit via back propagation  NCopyOutMin=[]  NCopyOutMax=[]  IntegratorContinuousStateAttributes=''  IntegratorStateMustResolveToSignalObject=off  IntegratorRTWStateStorageClass=Auto  FilterContinuousStateAttributes=''  FilterStateMustResolveToSignalObject=off  FilterRTWStateStorageClass=Auto  ParallelPVariant=InternalParameters  IdealPVariant=Disabled  IVariant=InternalParameters  DVariant=Disabled  IntegratorVariant=Discrete  SatVariant=Enabled  AWVariant=Passthrough  PCopyVariant=Disabled  TRVariant=Disabled  FdbkBlocksVariant=Forward  IdealPFdbkVariant=Disabled  SatFdbkVariant=Disabled  DerivativeFilterVariant=Disabled  NVariant=Disabled  NCopyVariant=Disabled_SignalSpec  FilterICVariant=Disabled  IntegratorICVariant=InternalICs  ExternalResetVariant=ExternalReset  TRSumVariant=Passthrough  SumFdbkVariant=Disabled  SumVariant=Sum_PI  TsampFilterVariant=InternalTs  TsampNgainVariant=Passthrough  TsampIntegralVariant=Disabled_SignalSpec  ExternalSaturationOutDataTypeStr=Inherit: Same as second input  DerivativeSourceVariant=Disabled  PreIntVariant=InternalPreInt
      settings: LibrarySourceBlock=simulink/Discrete/Discrete PID Controller
  Product : Product  RndMeth=Simplest  OutDataTypeStr=Inherit: Same as first input
  Product3 : Product  RndMeth=Simplest  OutDataTypeStr=Inherit: Same as first input
  Sqrt : Sqrt  RndMeth=Simplest
  Sum : Sum  Inputs=|+-
  Id_ref : Outport
  wires:
  Sqrt/1 -> Sum/2
  Add1/1 -> Sqrt/1
  Demux/2 -> Product3/2, Product3/1
  Delay One Step/1 -> Demux/1
  Product/1 -> Add1/1
  Constant/1 -> Sum/1
  Demux/1 -> Product/1, Product/2
  Discrete PID Controller/1 -> Id_ref/1
  Sum/1 -> Discrete PID Controller/1
  Product3/1 -> Add1/2
  vdq/1 -> Delay One Step/1
  Compare To Constant/1 -> Discrete PID Controller/2
  SpeedRef/1 -> Compare To Constant/1

== system mchp_acim_dsPIC33A/Control algorithm/Motor Control Application/FOC/VbyF ControlReference/Wrap_to_pi1 ==
  note: Subtract pi
  note: What's left after
      | division by 2pi
      | again
  note: Add pi
  note: This block limits the output angle between +/- π.
  note: What's left after
      | division by 2pi
  θ : Inport
  Bias : Bias  Bias=pi  SaturateOnIntegerOverflow=off
  Bias1 : Bias  Bias=-pi  SaturateOnIntegerOverflow=off
  Math Function : Math  Operator=mod  SignedPower=on
  Math Function1 : Math  Operator=mod  SignedPower=on
  load torque1 : Constant  Value=2*pi  OutDataTypeStr=single  SampleTime=Ts_mc
  θ (-π,π) : Outport  VectorParamsAs1DForOutWhenUnconnected=off
  wires:
  Bias1/1 -> θ (-π,π)/1
  Bias/1 -> Math Function/1
  load torque1/1 -> Math Function/2, Math Function1/2
  Math Function/1 -> Bias1/1
  θ/1 -> Math Function1/1
  Math Function1/1 -> Bias/1

== system mchp_acim_dsPIC33A/Control algorithm/Data Monitoring/SerialOutDrivers/codegen/SCI_Tx/Data ==
  Data : Inport
  Action Port : ActionPort  ActionPortLabel=else
  UART Tx : MCHP_Blockset/BUS UART/UART Tx  UART_REF=1  ORDERING=None  AllOrNothing=off  SampleTime=-1  MCHP_MASTERLINK=mchp_acim_dsPIC33A/MCHV-230VAC-1.5kW Development Board dsPIC33AK128MC106 MC DIM/Microchip Master  NSend_Input=off  UART_String=off  NSend_Output=off
      settings: SourceProductName=MPLAB Device Blocks for Simulink
  wires:
  Data/1 -> UART Tx/1

== system mchp_acim_dsPIC33A/Control algorithm/Data Monitoring/SerialOutDrivers/codegen/SCI_Tx/End ==
  Data : Inport
  Action Port : ActionPort  ActionPortLabel=elseif(u1 == u2)
  Mux : Mux  Inputs=2
  Start : Constant  Value=hex2dec('45')  OutDataTypeStr=uint8
  UART Tx : MCHP_Blockset/BUS UART/UART Tx  UART_REF=1  ORDERING=None  AllOrNothing=off  SampleTime=-1  MCHP_MASTERLINK=mchp_acim_dsPIC33A/MCHV-230VAC-1.5kW Development Board dsPIC33AK128MC106 MC DIM/Microchip Master  NSend_Input=off  UART_String=off  NSend_Output=off
      settings: SourceProductName=MPLAB Device Blocks for Simulink
  wires:
  Mux/1 -> UART Tx/1
  Data/1 -> Mux/1
  Start/1 -> Mux/2

== system mchp_acim_dsPIC33A/Control algorithm/Data Monitoring/SerialOutDrivers/codegen/SCI_Tx/Start ==
  Data : Inport
  Action Port : ActionPort  ActionPortLabel=if(u1 == 0)
  End : Constant  Value=hex2dec('53')  OutDataTypeStr=uint8
  Mux : Mux  Inputs=2
  UART Tx : MCHP_Blockset/BUS UART/UART Tx  UART_REF=1  ORDERING=None  AllOrNothing=off  SampleTime=-1  MCHP_MASTERLINK=mchp_acim_dsPIC33A/MCHV-230VAC-1.5kW Development Board dsPIC33AK128MC106 MC DIM/Microchip Master  NSend_Input=off  UART_String=off  NSend_Output=off
      settings: SourceProductName=MPLAB Device Blocks for Simulink
  wires:
  Mux/1 -> UART Tx/1
  Data/1 -> Mux/2
  End/1 -> Mux/1

== system mchp_acim_dsPIC33A/Control algorithm/Motor Control Application/FOC/Estimator Interface/BEMF-PLL Sensorless estimator1/Integrator ==
  In : Inport
  ResetTrigger : Inport  Port=2
  ResetThetaValue : Inport  Port=3
  " " : Gain  Gain=Ts_mc  ParamDataTypeStr=single  OutDataTypeStr=single
  Data Type Conversion1 : DataTypeConversion  OutDataTypeStr=fixdt(1,32,31)  SaturateOnIntegerOverflow=off  RndMeth=Floor
  Data Type Conversion2 : DataTypeConversion  OutDataTypeStr=fixdt(1,32,31)  SaturateOnIntegerOverflow=off  RndMeth=Floor
  Data Type Conversion3 : DataTypeConversion  OutDataTypeStr=fixdt(1,16,15)  SaturateOnIntegerOverflow=off  RndMeth=Floor
  Delay One Step1 : Delay  DelayLength=1  InitialConditionSource=Input port  InitialCondition=0  ExternalReset=Rising  SampleTime=Ts_mc
      settings: InputPortMap=u0,r5,p4
  PU : Gain  Gain=1/pi  ParamDataTypeStr=single  OutDataTypeStr=single
  PU1 : Gain  Gain=pi  ParamDataTypeStr=single  OutDataTypeStr=single
  PU2 : Gain  Gain=1/pi  ParamDataTypeStr=single  OutDataTypeStr=fixdt(1,32,31)
  Subtract3 : Sum  OutDataTypeStr=fixdt(1,32,31)
  theta : Outport
  wires:
  Data Type Conversion1/1 -> Subtract3/1
  Delay One Step1/1 -> Subtract3/2
  Data Type Conversion3/1 -> PU1/1
  " "/1 -> PU/1
  Subtract3/1 -> Data Type Conversion3/1, Delay One Step1/1
  PU/1 -> Data Type Conversion1/1
  PU1/1 -> theta/1
  In/1 -> " "/1
  ResetTrigger/1 -> Delay One Step1/2
  ResetThetaValue/1 -> PU2/1
  PU2/1 -> Data Type Conversion2/1
  Data Type Conversion2/1 -> Delay One Step1/3

== system mchp_acim_dsPIC33A/Control algorithm/Motor Control Application/FOC/Estimator Interface/BEMF-PLL Sensorless estimator1/LPF ==
  In1 : Inport
  Reset : Inport  Port=2
  Add1 : Sum
  Delay : Delay  DelayLength=1  ExternalReset=Rising
      settings: InputPortMap=u0,r5
  Gain1 : Gain  Gain=(Ts_mc/(Ts_mc+(1/(2*pi*160))))  OutDataTypeStr=single
  Subtract : Sum  Inputs=+-
  Out1 : Outport
  wires:
  Gain1/1 -> Add1/2
  Delay/1 -> Subtract/2, Add1/1
  Subtract/1 -> Gain1/1
  Add1/1 -> Delay/1, Out1/1
  In1/1 -> Subtract/1
  Reset/1 -> Delay/2

== system mchp_acim_dsPIC33A/Control algorithm/Motor Control Application/FOC/Estimator Interface/BEMF-PLL Sensorless estimator1/LPF1 ==
  In1 : Inport
  Reset : Inport  Port=2
  Add1 : Sum
  Delay : Delay  DelayLength=1  ExternalReset=Rising
      settings: InputPortMap=u0,r5
  Gain1 : Gain  Gain=(Ts_mc/(Ts_mc+(1/(2*pi*160))))  OutDataTypeStr=single
  Subtract : Sum  Inputs=+-
  Out1 : Outport
  wires:
  Reset/1 -> Delay/2
  In1/1 -> Subtract/1
  Add1/1 -> Out1/1, Delay/1
  Subtract/1 -> Gain1/1
  Delay/1 -> Add1/1, Subtract/2
  Gain1/1 -> Add1/2

== system mchp_acim_dsPIC33A/Control algorithm/Motor Control Application/FOC/Estimator Interface/BEMF-PLL Sensorless estimator1/LPF2 ==
  In1 : Inport
  Reset : Inport  Port=2
  Add1 : Sum
  Delay : Delay  DelayLength=1  ExternalReset=Rising
      settings: InputPortMap=u0,r5
  Gain1 : Gain  Gain=(Ts_mc/(Ts_mc+(1/(2*pi*SpeedFilterCutoff))))  OutDataTypeStr=single
  Subtract : Sum  Inputs=+-
  Out1 : Outport
  wires:
  Reset/1 -> Delay/2
  In1/1 -> Subtract/1
  Add1/1 -> Out1/1, Delay/1
  Subtract/1 -> Gain1/1
  Delay/1 -> Add1/1, Subtract/2
  Gain1/1 -> Add1/2

== system mchp_acim_dsPIC33A/Control algorithm/Motor Control Application/FOC/Estimator Interface/BEMF-PLL Sensorless estimator1/Slip speed estimator ==
  Iqs_ref : Inport
  Id_ref : Inport  Port=2
  Init : Inport  Port=3
  Add1 : Sum
  Constant : Constant  Value=(acim.Lm+acim.Llr)/acim.Rr  OutDataTypeStr=single  SampleTime=-1
  Delay : Delay  DelayLength=1  ExternalReset=Rising
      settings: InputPortMap=u0,r5
  Divide : Product  Inputs=*/
  Gain1 : Gain  Gain=Ts_mc/( Ts_mc + (acim.Lm+acim.Llr)/acim.Rr )  OutDataTypeStr=single
  Product : Product
  Subtract : Sum  Inputs=+-
  slip : Outport
  wires:
  Id_ref/1 -> Subtract/1
  Add1/1 -> Product/1, Delay/1
  Subtract/1 -> Gain1/1
  Delay/1 -> Add1/1, Subtract/2
  Gain1/1 -> Add1/2
  Iqs_ref/1 -> Divide/1
  Constant/1 -> Product/2
  Product/1 -> Divide/2
  Divide/1 -> slip/1
  Init/1 -> Delay/2

== system mchp_acim_dsPIC33A/Control algorithm/Motor Control Application/FOC/Estimator Interface/Speed & postion interface (sensored)/Wrap_to_pi1 ==
  note: Subtract pi
  note: What's left after
      | division by 2pi
      | again
  note: Add pi
  note: This block limits the output angle between +/- π.
  note: What's left after
      | division by 2pi
  θ : Inport
  Bias : Bias  Bias=pi  SaturateOnIntegerOverflow=off
  Bias1 : Bias  Bias=-pi  SaturateOnIntegerOverflow=off
  Math Function : Math  Operator=mod  SignedPower=on
  Math Function1 : Math  Operator=mod  SignedPower=on
  load torque1 : Constant  Value=2*pi  OutDataTypeStr=single  SampleTime=Ts_mc
  θ (-π,π) : Outport  VectorParamsAs1DForOutWhenUnconnected=off
  wires:
  Bias1/1 -> θ (-π,π)/1
  Bias/1 -> Math Function/1
  load torque1/1 -> Math Function/2, Math Function1/2
  Math Function/1 -> Bias1/1
  θ/1 -> Math Function1/1
  Math Function1/1 -> Bias/1

== system mchp_acim_dsPIC33A/Control algorithm/Motor Control Application/FOC/Generate Id reference/Inverse Speed based Flux Weakening/If Action Subsystem ==
  speedRef : Inport
  Action Port : ActionPort  ActionPortLabel=if((u1 > 0))
  Divide : Product  Inputs=**/
  Saturation : Saturate  UpperLimit=acim.Id0  LowerLimit=acim.Id0/2
  id : Constant  Value=acim.Id0  OutDataTypeStr=single  SampleTime=Ts_mc
  id1 : Constant  Value=acim.N_rated*0.9  OutDataTypeStr=single  SampleTime=Ts_mc
  id_ref : Outport
  wires:
  speedRef/1 -> Divide/3
  id/1 -> Divide/1
  id1/1 -> Divide/2
  Divide/1 -> Saturation/1
  Saturation/1 -> id_ref/1

== system mchp_acim_dsPIC33A/Control algorithm/Motor Control Application/FOC/Generate Id reference/Inverse Speed based Flux Weakening/If Action Subsystem1 ==
  Action Port : ActionPort  ActionPortLabel=else
  id : Constant  Value=acim.Id0  OutDataTypeStr=single  SampleTime=Ts_mc
  id_ref : Outport
  wires:
  id/1 -> id_ref/1

== stateflow chart mchp_acim_dsPIC33A/Control algorithm/Motor Control Application/appState State Machine/System Control ==
  settings: updateMethod=DISCRETE  sampleTime=Ts_mc
  state Cmd_Wait
    entry:
    MC1appState = appState.CMD_WAIT;
    CurrentOffsetCalib = false;
    CurrentOffsetFlag_out = true;
    Init = 1;
  state Init
    entry:
    MC1appState = appState.INIT;
    Init = 0;
    stop = 0;
  state Offset_Meas
    entry:
    MC1appState = appState.OFFSET_MEAS;
    CurrentOffsetCalib = true;
  state Openloop
    entry:
    MC1appState= appState.VF_OPEN_LOOP;
  state FOC_closed_loop
    entry:
    MC1appState= appState.FOC_CLOSED_LOOP;
  state Stopping
    entry:
    stop = 1;
  state Stop
    entry:
    MC1appState = appState.STOP;
  Init -> Cmd_Wait [order 2] : [CurrOffsetFlag == true]
  (default) -> Init
  Cmd_Wait -> (junction 182) : [RunCmd == true]{Init=0}
  (junction 182) -> FOC_closed_loop [order 1] : [operationMode==1]
  (junction 182) -> Openloop [order 2]
  Init -> Offset_Meas [order 1] : [CurrOffsetFlag == false]
  Offset_Meas -> Cmd_Wait : [after(0.2,sec)]
  Stop -> Init
  Openloop -> FOC_closed_loop [order 2] : [(operationMode==2)&&(SpeedRef > OL_SPEED)]
  Openloop -> Stopping [order 1] : [RunCmd == false]
  FOC_closed_loop -> Stopping : [RunCmd == false]
  Stopping -> Stop : [SpeedRef <= Min_speed]
  data: RunCmd input; SpeedRef input; operationMode input; OL_SPEED input; MC1appState output Enum: appState =appState.INIT; Init output single; CurrentOffsetCalib output; Estim_Speed input; Min_speed input; CurrOffsetFlag input boolean; CurrentOffsetFlag_out output; stop output single
